simulink model "SistemaCAS_v6_2"  (R2014a)
settings: Solver=ode45  StartTime=0.0  StopTime=10  RelTol=1e-3
libraries: simulink x1, dspsrcs4 x1
settings Model: Creator=andre  LastModifiedBy=andre

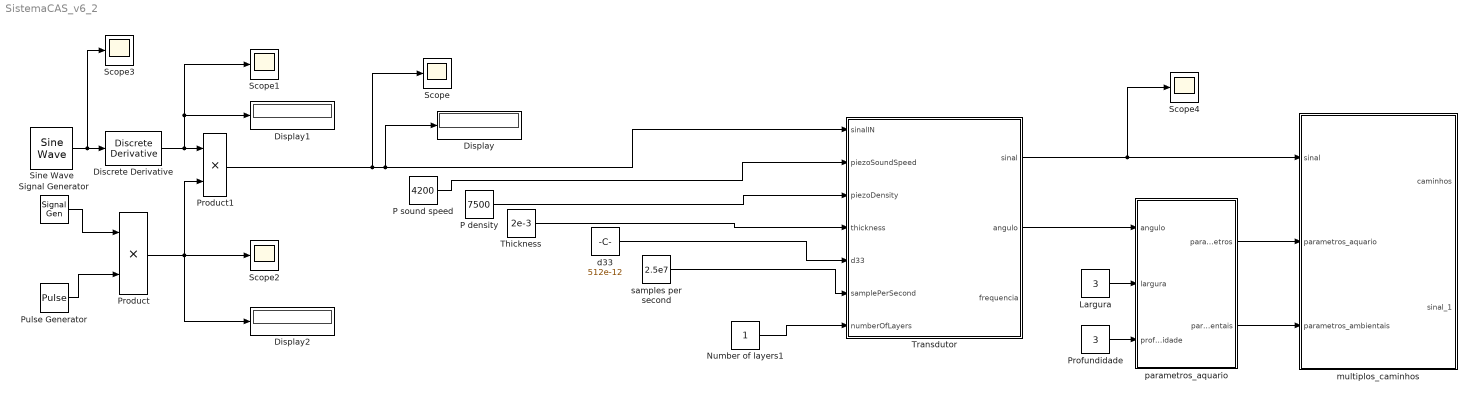
== system SistemaCAS_v6_2 ==
  Discrete Derivative : simulink/Discrete/Discrete Derivative  gainval=1.0  ICPrevScaledInput=0.0  InputProcessing=Inherited  OutMin=[]  OutMax=[]  OutDataType=fixdt(1, 16)  OutScaling=2^-10  DoSatur=off
  Display : Display
  Display1 : Display
  Display2 : Display
  Largura : Constant  Value=3
  Number of layers1 : Constant
  P density : Constant  Value=7500
  P sound speed : Constant  Value=4200
  Product : Product
  Product1 : Product
  Profundidade : Constant  Value=3
  Pulse Generator : DiscretePulseGenerator  Period=10
  Scope{,1..4} (5 alike) : Scope
      Scope2 settings: SaveName=ScopeData2
      Scope3 settings: SaveName=ScopeData3
      Scope4 settings: SaveName=ScopeData4
  Signal Generator : SignalGenerator  Amplitude=4  Frequency=10  Units=rad/sec
  Sine Wave : dspsrcs4/Sine Wave  Amplitude=10  Frequency=1  Phase=0  SampleMode=Discrete  OutComplex=Real  CompMethod=Trigonometric fcn  TableSize=Speed  SampleTime=1/1000  SamplesPerFrame=1  ResetState=Restart at time zero  dataType=double  wordLen=16  udDataType=sfix(16)  fracBitsMode=Best precision  numFracBits=15  OutDataTypeStr=double  LastOutDataTypeStr=double
  Thickness : Constant  Value=2e-3
  Transdutor : MATLAB Function  TreatAsAtomicUnit=on
  d33 : Constant  Value=512e-12
  multiplos_caminhos : MATLAB Function  TreatAsAtomicUnit=on
  parametros_aquario : MATLAB Function  TreatAsAtomicUnit=on
  samples per second : Constant  Value=2.5e7
  wires:
  Discrete Derivative/1 -> Display1/1, Scope1/1, Product1/1
  Signal Generator/1 -> Product/1
  Product/1 -> Display2/1, Scope2/1, Product1/2
  Sine Wave/1 -> Scope3/1, Discrete Derivative/1
  Pulse Generator/1 -> Product/2
  d33/1 -> Transdutor/5(d33)
  samples per second/1 -> Transdutor/6(samplePerSecond)
  Product1/1 -> Transdutor/1(sinalIN), Display/1, Scope/1
  P sound speed/1 -> Transdutor/2(piezoSoundSpeed)
  P density/1 -> Transdutor/3(piezoDensity)
  Thickness/1 -> Transdutor/4(thickness)
  Number of layers1/1 -> Transdutor/7(numberOfLayers)
  Largura/1 -> parametros_aquario/2(largura)
  Profundidade/1 -> parametros_aquario/3(profundidade)
  Transdutor/2(angulo) -> parametros_aquario/1(angulo)
  parametros_aquario/1(parametros) -> multiplos_caminhos/2(parametros_aquario)
  Transdutor/1(sinal) -> Scope4/1, multiplos_caminhos/1(sinal)
  parametros_aquario/2(parametros_ambientais) -> multiplos_caminhos/3(parametros_ambientais)

== matlab function SistemaCAS_v6_2/Transdutor ==
  data: sinalIN input; sinal output; piezoSoundSpeed input; piezoDensity input; thickness input; d33 input; samplePerSecond input; numberOfLayers input; angulo output; frequencia output
function [sinal, angulo, frequencia] = projetor(sinalIN, piezoSoundSpeed, piezoDensity, thickness, d33, samplePerSecond, numberOfLayers)


%-------------------------------------------------------------------------
% Sinal 
%-------------------------------------------------------------------------
sinal=sinalIN;

%-------------------------------------------------------------------------
% Ângulo de diretividade do transdutor calculado no COMSOL (rad)
%-------------------------------------------------------------------------
angulo = pi/3;            % (ex.: 60º = pi/3 rad)

%-------------------------------------------------------------------------
% Frequência do Sinal (kHz)
%-------------------------------------------------------------------------
frequencia = 1:2:2000;

== matlab function SistemaCAS_v6_2/multiplos_caminhos ==
  data: sinal input; caminhos output; sinal_1 output; parametros_aquario input; parametros_ambientais input
function [caminhos,sinal_1] = multiplos_caminhos(sinal, parametros_aquario,parametros_ambientais)
%Definir as distâncias de cada caminho
%Atrasar o sinal de cada caminho
%Enviar a distância e o sinal de cada caminho ()

w = parametros_aquario(1);
l = parametros_aquario(2);
d = parametros_aquario(3);

T = parametros_ambientais(1);
S = parametros_ambientais(2);
pH = parametros_ambientais(3);

%%%%%%  Bloco multipath  %%%%%%

%-------------------------------------------------------------------------
%Definindo as distâncias de cada caminho do multipath
%-------------------------------------------------------------------------
% caminho_1 = caminho refletido na superfície
% caminho_2 = caminho refletido na lateral de trás
% caminho_3 = caminho direto
% caminho_4 = caminho refletido na lateral da frente
% caminho_5 = caminho refletido no fundo
caminhos = [0 0 0 0 0];
caminhos(1) = sqrt(d^2 + l^2);
caminhos(2) = sqrt(w^2 + l^2);
caminhos(3) = l;
caminhos(4) = caminhos(2);
caminhos(5) = caminhos(1);

%-------------------------------------------------------------------------
%Definindo a profundidade média para cada caminho
%-------------------------------------------------------------------------
D = [0 0 0 0 0];
D(1) = mean([d/2,0]);
D(2) = d/2;
D(3) = d/2;
D(4) = d/2;
D(5) = mean([d,d/2]);

%-------------------------------------------------------------------------
%Velocidade do som na água (m/s)
%-------------------------------------------------------------------------
C = [0 0 0 0 0];
for i = 1:5 %5 caminhos
    c = 1448.96 + 4.591*T - 5.304*(10^(-2))*(T^(2))...
        + 2.374*(10^(-4))*(T^(3)) + 1.340*(S-35) + 1.630*(10^(-2))*D(i)...
        + 1.675*(10^(-7))*(D(i)^(2)) - 1.025*(10^(-2))*T*(S-35)...
        - 7.139*(10^(-13))*T*(D(i)^(3));
    
    %Conversão de (m/s) para (cm/s)
    C(i)=c*100;
end

%-------------------------------------------------------------------------
% Definindo os atrasos de cada caminho do multipath através da equação de
% velocidade de propagação do som na água
%-------------------------------------------------------------------------

% atraso é o tempo que o caminho leva

atraso1 = D(1)/C(1);
atraso2 = D(2)/C(2);
atraso3 = D(3)/C(3); % caminho direto não tem atraso
atraso4 = D(4)/C(4);
atraso5 = D(5)/C(5);

%-------------------------------------------------------------------------
% Atrasar os sinais de cada caminho
%-------------------------------------------------------------------------

% discretiza o sinal
%sysd = c2d(sys,Ts)
    
Y = fft(sinal);
Y1 = Y*exp(-atraso1);
sinal_1 = ifft(Y1);
% Y2 = Y*exp(-atraso2);
% sinal_2 = ifft(Y2);
% Y3 = Y*exp(-atraso3);
% sinal_3 = ifft(Y3);
% Y4 = Y*exp(-atraso4);
% sinal_4 = ifft(Y4);
% Y5 = Y*exp(-atraso5);
% sinal_5 = ifft(Y5);


% sinal_1 = sinal + atraso1; 
sinal_2 = sinal + atraso2;
sinal_3 = sinal + atraso3;
sinal_4 = sinal + atraso4;
sinal_5 = sinal + atraso5;

== matlab function SistemaCAS_v6_2/parametros_aquario ==
  data: angulo input; largura input; profundidade input; parametros output; parametros_ambientais output
function [parametros,parametros_ambientais] = parametros_aquario(angulo,largura,profundidade)
% consideraçoes para os parâmetros do aquário
% 1. emissor e receptor estão alinhados ( largura(x) e profundidade(z)
% iguais, só muda o comprimento (y)
% 2. o comprimento do aquario (L) é ideal para acontecer uma reflexão completa
% com o angulo de diretividade (que é o maior angulo possível do lóbulo 
% principal utilizando o transdutor piezoeletrico escolhido)
% 3. para facilitar os cálculos de do comprimento ideal, utilizamos largura
% igual profundidade (D = W)

% considerações sobre a simulação
% 1. serão considerados somente os caminhos do angulo de diretividade e o
% caminho direto (5 caminhos: um direto, dois que refletem nas laterais, e
% dois que refletem na superfície e o fundo
% 2. a reflexão será considerada reflexão completa com um eco (sem perdas 
% de energia ou refraçao)

%-------------------------------------------------------------------------
%Parâmetros do Aquário definidos anteriormente
%-------------------------------------------------------------------------
w = largura;                  % largura (eixo x)
d = profundidade;             % profundidade do aquário (eixo z) 
l = w/sin(angulo/2);      % comprimento do aquário calculado utilizando o angulo de diretividade (eixo y)
% l(éle) é a distancia ideal para acontecer uma reflexão completa
parametros = [w,l,d];


%-------------------------------------------------------------------------
% Valores dos parâmetros do meio subaquático 
%-------------------------------------------------------------------------
T = 32;                 % Temperatura (°C)
S = 1;                  % Salinidade (ppt)
pH = 7.2;               % acidêz da água - pH (potencial hidrogeniônico)
parametros_ambientais = [T, S, pH];
